simulink model "USBamp_signalCheck"  (R2015a)
settings: Solver=ode45  StartTime=0.0  StopTime=Inf  RelTol=1e-3
undefined symbols (not defined in the file or in its folder): currentCFG_USBamp_online_UB, UB
libraries: Tools x1, gtecHighspeedLib x1, gUSBamplib x1
settings Model: Creator=Co  LastModifiedBy=Co
settings OptimizationCC: BlockReduction=off

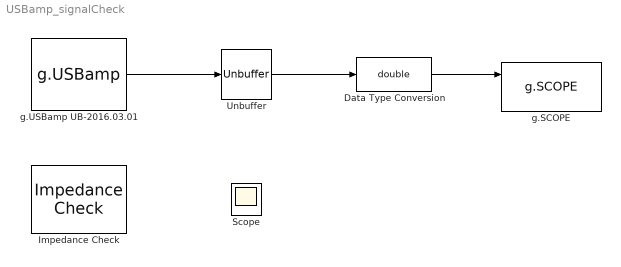
== system USBamp_signalCheck ==
  Data Type Conversion : DataTypeConversion  OutDataTypeStr=double
  Impedance Check : Tools/Impedance Check
  Scope : Scope
  Unbuffer : Unbuffer  SampleBasedProcessing=Same as frame based
  g.SCOPE : gtecHighspeedLib/g.SCOPE
  g.USBamp UB-2016.03.01 : gUSBamplib/g.USBamp  cfg=currentCFG_USBamp_online_UB-2016.03.01.cfg  snr=UB-2016.03.01
  wires:
  g.USBamp UB-2016.03.01/1 -> Unbuffer/1
  Unbuffer/1 -> Data Type Conversion/1
  Data Type Conversion/1 -> g.SCOPE/1
